simulink model "seond_copy_of_Rotary_system_h_bridge_23a"  (R2023a)
settings: Solver=ode4  StartTime=0.0  StopTime=0.25  FixedStep=1e-6  RelTol=1e-3
InitFcn:
  | %% Parameters
  | 
  | param = struct();
  | 
  | % Volume of chambers
  | param.V1_0 = 1e-3;
  | param.V2_0 = 20e-6;
  | 
  | % Pressure rails
  | param.P_H = 20e6;
  | param.P_M = 10e6;
  | 
  | % Valve things
  | param.max_Avt = 0.5*0.25*pi*(20e-3)^2;
  | param.Cd = 0.6;
  | 
  | % Fluid properties
  | param.beta = 1.8e9;
  | param.rho = 870;
  | 
  | % Electric motor stuff
  | param.Kt = 70.5e-3;
  | param.Ke = 70.5e-3;
  | param.J_elec = 3000e-7;
  | 
  | % Pump things
  | param.J_hyd = 3000e-7;
  | param.hyd_D = 1.6e-6;    % In cc/rev
  | 
  | % Simulation time
  | T = 1.2;
settings Model: Creator=user  LastModifiedBy=ibrah408

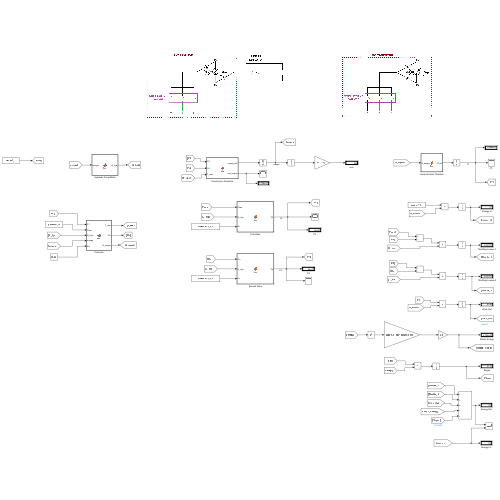
[thumbnail: Simulink's stored preview of the top-level diagram]
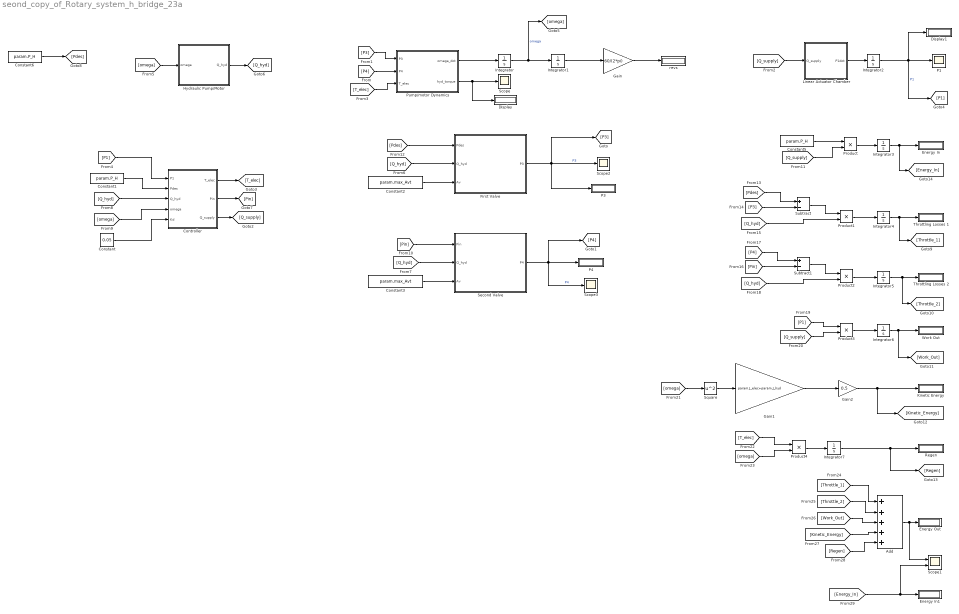
== system seond_copy_of_Rotary_system_h_bridge_23a ==
  Add : Sum  Inputs=+++++
  Constant : Constant  Value=0.05
  Constant1 : Constant  Value=param.P_H
  Constant2 : Constant  Value=param.max_Avt
  Constant3 : Constant  Value=param.max_Avt
  Constant5 : Constant  Value=param.P_H
  Constant6 : Constant  Value=param.P_H
  Controller : MATLAB Function  TreatAsAtomicUnit=on
  Display : Display
  Display1 : Display
  Energy In : Display
  Energy In1 : Display
  Energy Out : Display
  First Valve : MATLAB Function  TreatAsAtomicUnit=on
  Gain : Gain  Gain=60/(2*pi)
  Gain1 : Gain  Gain=param.J_elec+param.J_hyd
  Gain2 : Gain  Gain=0.5
  Hydraulic Pump/Motor : MATLAB Function  TreatAsAtomicUnit=on
  Integrator{,1,3..7} (7 alike) : Integrator
  Integrator2 : Integrator  InitialCondition=param.P_M
  Kinetic Energy : Display
  Linear Actuator Chamber : MATLAB Function  TreatAsAtomicUnit=on
  P1 : Scope
  P3 : Display
  P4 : Display
  Product{,1..4} (5 alike) : Product
  Pump/motor Dynamics : MATLAB Function  TreatAsAtomicUnit=on
  Regen : Display
  Scope : Scope
  Scope1 : Scope  NumInputPorts=2
  Scope2 : Scope
  Scope3 : Scope
  Second Valve : MATLAB Function  TreatAsAtomicUnit=on
  Square : Math  Operator=square
  Subtract : Sum  Inputs=+-
  Subtract1 : Sum  Inputs=+-
  Throttling Losses 1 : Display
  Throttling Losses 2 : Display
  Work Out : Display
  revs : Display
  wires:
  Pump/motor Dynamics/1(omega_dot) -> Integrator/1
  Integrator/1 -> [omega], Integrator1/1  "omega"
  Integrator1/1 -> Gain/1
  Gain/1 -> revs/1
  Constant2/1 -> First Valve/3(Av)
  Constant3/1 -> Second Valve/3(Av)
  Linear Actuator Chamber/1(P1dot) -> Integrator2/1
  Integrator2/1 -> [P1], Display1/1, P1/1  "P1"
  First Valve/1(P3) -> Scope2/1, [P3], P3/1  "P3"
  Second Valve/1(P4) -> Scope3/1, [P4], P4/1  "P4"
  Constant/1 -> Controller/5(Kd)
  [P4] -> Pump/motor Dynamics/2(P4)
  [P3] -> Pump/motor Dynamics/1(P3)
  [Pdes] -> First Valve/1(Pdes)
  Controller/3(Q_supply) -> [Q_supply]
  [Q_supply] -> Linear Actuator Chamber/1(Q_supply)
  Controller/1(T_elec) -> [T_elec]
  [T_elec] -> Pump/motor Dynamics/3(T_elec)
  [P1] -> Controller/1(P1)
  Constant1/1 -> Controller/2(Pdes)
  [omega] -> Hydraulic Pump/Motor/1(omega)
  Hydraulic Pump/Motor/1(Q_hyd) -> [Q_hyd]
  [Q_hyd] -> First Valve/2(Q_hyd)
  [Q_hyd] -> Second Valve/2(Q_hyd)
  [Q_hyd] -> Controller/3(Q_hyd)
  [omega] -> Controller/4(omega)
  Controller/2(Pin) -> [Pin]
  [Pin] -> Second Valve/1(Pin)
  [Q_supply] -> Product/2
  Constant5/1 -> Product/1
  Product/1 -> Integrator3/1
  Integrator3/1 -> [Energy_In], Energy In/1
  Subtract/1 -> Product1/1
  Constant6/1 -> [Pdes]
  [Pdes] -> Subtract/1
  [P3] -> Subtract/2
  [Q_hyd] -> Product1/2
  Product1/1 -> Integrator4/1
  Product2/1 -> Integrator5/1
  [Q_hyd] -> Product2/2
  Subtract1/1 -> Product2/1
  Integrator5/1 -> [Throttle_2], Throttling Losses 2/1
  [P4] -> Subtract1/1
  [Pin] -> Subtract1/2
  [Q_supply] -> Product3/2
  [P1] -> Product3/1
  Product3/1 -> Integrator6/1
  Integrator6/1 -> [Work_Out], Work Out/1
  [omega] -> Square/1
  Square/1 -> Gain1/1
  Gain1/1 -> Gain2/1
  Gain2/1 -> Kinetic Energy/1, [Kinetic_Energy]
  Pump/motor Dynamics/2(hyd_torque) -> Display/1, Scope/1
  [T_elec] -> Product4/1
  [omega] -> Product4/2
  Product4/1 -> Integrator7/1
  Integrator7/1 -> [Regen], Regen/1
  Integrator4/1 -> [Throttle_1], Throttling Losses 1/1
  [Throttle_1] -> Add/1
  [Throttle_2] -> Add/2
  [Work_Out] -> Add/3
  [Kinetic_Energy] -> Add/4
  [Regen] -> Add/5
  Add/1 -> Scope1/1, Energy Out/1
  [Energy_In] -> Scope1/2, Energy In1/1

== matlab function seond_copy_of_Rotary_system_h_bridge_23a/Pump//motor Dynamics ==
  data: omega_dot output; P3 input; P4 input; param parameter; T_elec input; hyd_torque output
function [omega_dot, hyd_torque] = fcn(P3, P4, param, T_elec)

hyd_torque = (param.hyd_D/(2*pi))*(P3-P4);
omega_dot = (1/(param.J_elec+param.J_hyd))*(hyd_torque - T_elec);

== matlab function seond_copy_of_Rotary_system_h_bridge_23a/Hydraulic Pump//Motor ==
  data: Q_hyd output; omega input; param parameter
function Q_hyd   = fcn(omega, param)

Q_hyd = (param.hyd_D/(2*pi))*omega;

== matlab function seond_copy_of_Rotary_system_h_bridge_23a/First Valve ==
  data: Pdes input; P3 output; Q_hyd input; Av input; param parameter
function P3 = fcn(Pdes, Q_hyd, Av, param)

K = param.Cd*Av*sqrt(2/param.rho);

P3 = Pdes - (Q_hyd/K)^2;

== matlab function seond_copy_of_Rotary_system_h_bridge_23a/Second Valve ==
  data: Pin input; P4 output; Q_hyd input; Av input; param parameter
function P4 = fcn(Pin, Q_hyd, Av, param)

K = param.Cd*Av*sqrt(2/param.rho);
P4 = Pin + (Q_hyd/K)^2;

== matlab function seond_copy_of_Rotary_system_h_bridge_23a/Linear Actuator Chamber ==
  data: P1dot output; Q_supply input; param parameter
function P1dot = fcn(Q_supply, param)

P1dot = (param.beta/param.V1_0)*(Q_supply);

== matlab function seond_copy_of_Rotary_system_h_bridge_23a/Controller ==
  data: P1 input; Pdes input; Q_hyd input; T_elec output; Pin output; Q_supply output; omega input; Kd input
function [T_elec, Pin, Q_supply] = fcn(P1, Pdes, Q_hyd, omega, Kd)

if abs(P1-Pdes)<1e4
    T_elec = Kd*omega;
    Pin = Pdes;
    Q_supply = 0;
else
    T_elec = 0;
    Pin = P1;
    Q_supply = Q_hyd;
end
